simulink model "CntctrCtrl"  (R2023b)
settings: Solver=VariableStepAuto  StartTime=0.0  StopTime=10.0  RelTol=1e-3
settings Model: Creator=OWNER  LastModifiedBy=OWNER

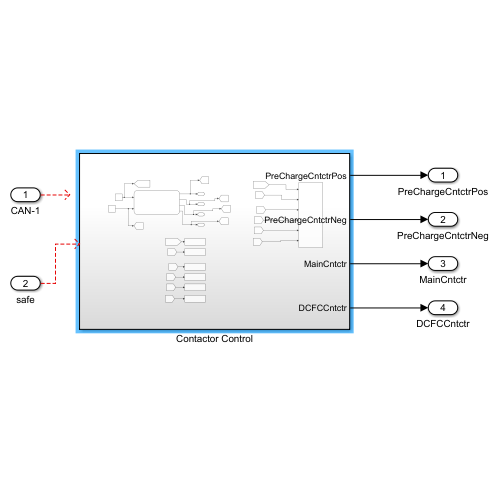
[thumbnail: Simulink's stored preview of the top-level diagram]
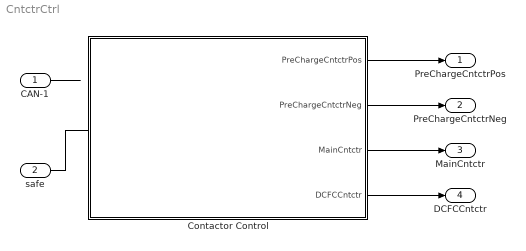
== system CntctrCtrl ==
  CAN-1 : Inport
  safe : Inport  Port=2
  Contactor Control : Subsystem
  PreChargeCntctrPos : Outport
  PreChargeCntctrNeg : Outport  Port=2
  MainCntctr : Outport  Port=3
  DCFCCntctr : Outport  Port=4
  wires:
  Contactor Control/4(DCFCCntctr) -> DCFCCntctr/1
  Contactor Control/1(PreChargeCntctrPos) -> PreChargeCntctrPos/1
  Contactor Control/2(PreChargeCntctrNeg) -> PreChargeCntctrNeg/1
  safe/1 -> ?
  Contactor Control/3(MainCntctr) -> MainCntctr/1
  CAN-1/1 -> ?

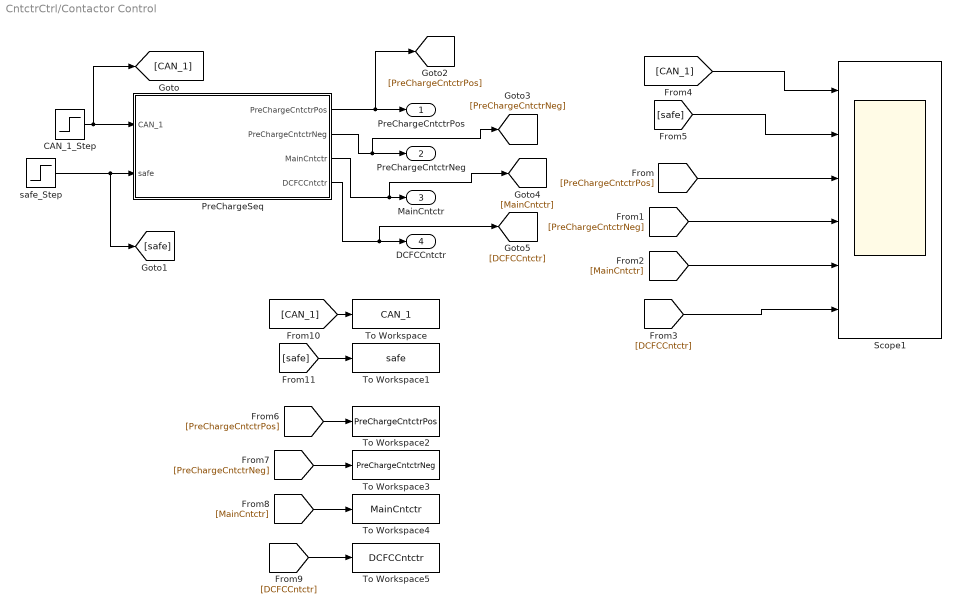
== system CntctrCtrl/Contactor Control ==
  CAN_1_Step : Step  After=2  SampleTime=0
  PreChargeSeq : Stateflow chart  TreatAsAtomicUnit=on
  Scope1 : Scope  NumInputPorts=6
  To Workspace : ToWorkspace  VariableName=CAN_1  SaveFormat=Timeseries  SampleTime=-1
  To Workspace1 : ToWorkspace  VariableName=safe  SaveFormat=Timeseries  SampleTime=-1
  To Workspace2 : ToWorkspace  VariableName=PreChargeCntctrPos  SaveFormat=Timeseries  SampleTime=-1
  To Workspace3 : ToWorkspace  VariableName=PreChargeCntctrNeg  SaveFormat=Timeseries  SampleTime=-1
  To Workspace4 : ToWorkspace  VariableName=MainCntctr  SaveFormat=Timeseries  SampleTime=-1
  To Workspace5 : ToWorkspace  VariableName=DCFCCntctr  SaveFormat=Timeseries  SampleTime=-1
  safe_Step : Step  Time=5  Before=1  After=0  SampleTime=0
  PreChargeCntctrPos : Outport
  PreChargeCntctrNeg : Outport  Port=2
  MainCntctr : Outport  Port=3
  DCFCCntctr : Outport  Port=4
  wires:
  CAN_1_Step/1 -> [CAN_1], PreChargeSeq/1(CAN_1)
  PreChargeSeq/1(PreChargeCntctrPos) -> [PreChargeCntctrPos], PreChargeCntctrPos/1
  safe_Step/1 -> PreChargeSeq/2(safe), [safe]
  PreChargeSeq/4(DCFCCntctr) -> [DCFCCntctr], DCFCCntctr/1
  PreChargeSeq/3(MainCntctr) -> [MainCntctr], MainCntctr/1
  PreChargeSeq/2(PreChargeCntctrNeg) -> [PreChargeCntctrNeg], PreChargeCntctrNeg/1
  [CAN_1] -> Scope1/1
  [PreChargeCntctrPos] -> Scope1/3
  [PreChargeCntctrNeg] -> Scope1/4
  [safe] -> Scope1/2
  [MainCntctr] -> Scope1/5
  [DCFCCntctr] -> Scope1/6
  [CAN_1] -> To Workspace/1
  [safe] -> To Workspace1/1
  [PreChargeCntctrPos] -> To Workspace2/1
  [PreChargeCntctrNeg] -> To Workspace3/1
  [MainCntctr] -> To Workspace4/1
  [DCFCCntctr] -> To Workspace5/1

== stateflow chart CntctrCtrl/Contactor Control/PreChargeSeq ==
  state PreChargeSeqInitialization
    entry:
    PreChargeCntctrPos = 0;
    PreChargeCntctrNeg = 0;
    MainCntctr = 0;
    DCFCCntctr = 0;
  state PreChargeSeqCharging
    state MainAndDCFCClosed
      entry:
      PreChargeCntctrPos = 0;
      PreChargeCntctrNeg = 0;
      MainCntctr = 1;
      DCFCCntctr = 1;
  state PreChargeSeqDischarging
    state PreChargeCntctrClosed
      entry:
      PreChargeCntctrPos = 1;
      PreChargeCntctrNeg = 1;
      MainCntctr = 0;
      DCFCCntctr = 0;
    state MainCntctrClosed
      entry:
      PreChargeCntctrPos = 1;
      PreChargeCntctrNeg = 1;
      MainCntctr = 1;
      DCFCCntctr = 0;
    state PreChargeCntctrOpen
      entry:
      PreChargeCntctrPos = 0;
      PreChargeCntctrNeg = 0;
      MainCntctr = 1;
      DCFCCntctr = 0;
    (default) -> PreChargeCntctrClosed
    PreChargeCntctrClosed -> MainCntctrClosed : after(100,msec)
    MainCntctrClosed -> PreChargeCntctrOpen : after(1.2, sec)
  state Fault
    entry:
    PreChargeCntctrPos = 0;
    PreChargeCntctrNeg = 0;
    MainCntctr = 0;
    DCFCCntctr = 0;
  (default) -> PreChargeSeqInitialization
  PreChargeSeqInitialization -> PreChargeSeqDischarging [order 1] : [CAN_1 == 1 && safe == 1]
  PreChargeSeqInitialization -> PreChargeSeqCharging [order 2] : [CAN_1 == 2 && safe == 1]
  PreChargeSeqDischarging -> Fault : [safe == 0]
  PreChargeSeqCharging -> Fault : [safe == 0]
  data: CAN_1 input; safe input; PreChargeCntctrPos output; PreChargeCntctrNeg output; MainCntctr output; DCFCCntctr output
